simulink model "teste_isolado"  (R2025b)
settings: Solver=VariableStepAuto  StartTime=0.0  StopTime=10  FixedStep=1e-9  MaxStep=5e-6  RelTol=1e-8
undefined symbols (not defined in the file or in its folder): magnitude
libraries: eeTransforms x1, simulink x1
settings Model: Creator=victo  LastModifiedBy=gilbr

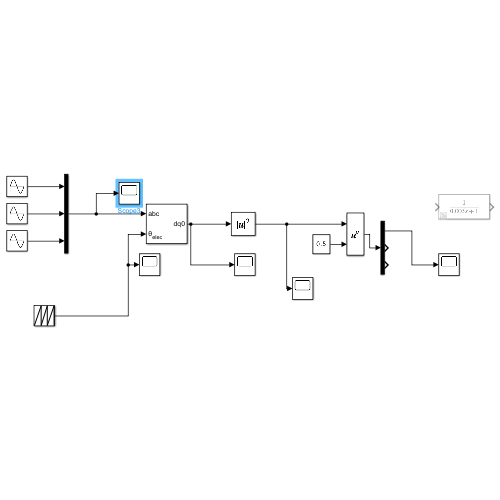
[thumbnail: Simulink's stored preview of the top-level diagram]
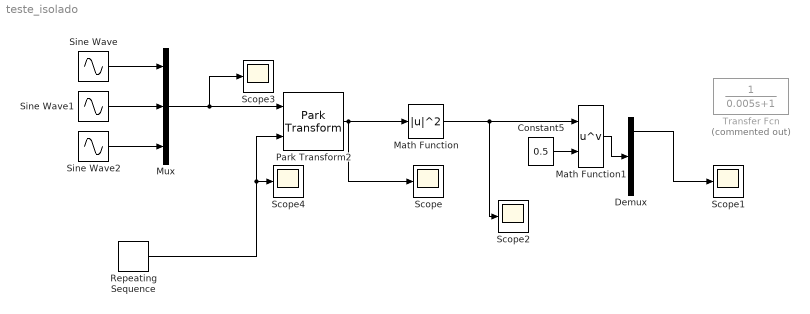
== system teste_isolado ==
  Constant5 : Constant  Value=0.5
  Demux : Demux  Outputs=3
  Math Function : Math  Operator=magnitude^2
  Math Function1 : Math  Operator=pow
  Mux : Mux  Inputs=3
  Park Transform2 : eeTransforms/Park Transform  AxisAlignment=Q-axis  PowerInvariant=off
  Repeating Sequence : simulink/Sources/Repeating Sequence  rep_seq_t=[0 1/60]  rep_seq_y=[0 2*pi]
  Scope{,1..4} (5 alike) : Scope
      Scope settings: ActiveDisplayYMinimum=-1.2500000000000016  ActiveDisplayYMaximum=1.2500000000000007  DataLoggingVariableName=ScopeData22
      Scope1 settings: ActiveDisplayYMinimum=0.99999999999995026  ActiveDisplayYMaximum=1.0000000000000497
      Scope2 settings: ActiveDisplayYMinimum=-0.12500000000001008  ActiveDisplayYMaximum=1.125000000000091  DataLoggingVariableName=ScopeData23
      Scope3 settings: ActiveDisplayYMinimum=-1.25  ActiveDisplayYMaximum=1.25
      Scope4 settings: ActiveDisplayYMinimum=0.40731742722113662  ActiveDisplayYMaximum=6.6103479493723007  DataLoggingVariableName=ScopeData2
  Sine Wave : Sin  Frequency=2*pi*60  SampleTime=0
  Sine Wave1 : Sin  Frequency=2*pi*60  Phase=-2*pi/3  SampleTime=0
  Sine Wave2 : Sin  Frequency=2*pi*60  Phase=2*pi/3  SampleTime=0
  Transfer Fcn : TransferFcn  Commented=on  Denominator=[0.005 1]
  wires:
  Mux/1 -> Scope3/1, Park Transform2/1
  Park Transform2/1 -> Math Function/1, Scope/1
  Math Function/1 -> Math Function1/1, Scope2/1
  Constant5/1 -> Math Function1/2
  Sine Wave/1 -> Mux/1
  Sine Wave1/1 -> Mux/2
  Sine Wave2/1 -> Mux/3
  Repeating Sequence/1 -> Scope4/1, Park Transform2/2
  Math Function1/1 -> Demux/1
  Demux/1 -> Scope1/1
